simulink model "completo"  (R2014b)
settings: Solver=ode23t  StartTime=0.0  StopTime=10.0  RelTol=1e-3
settings Model: Creator=Javi  LastModifiedBy=Javi

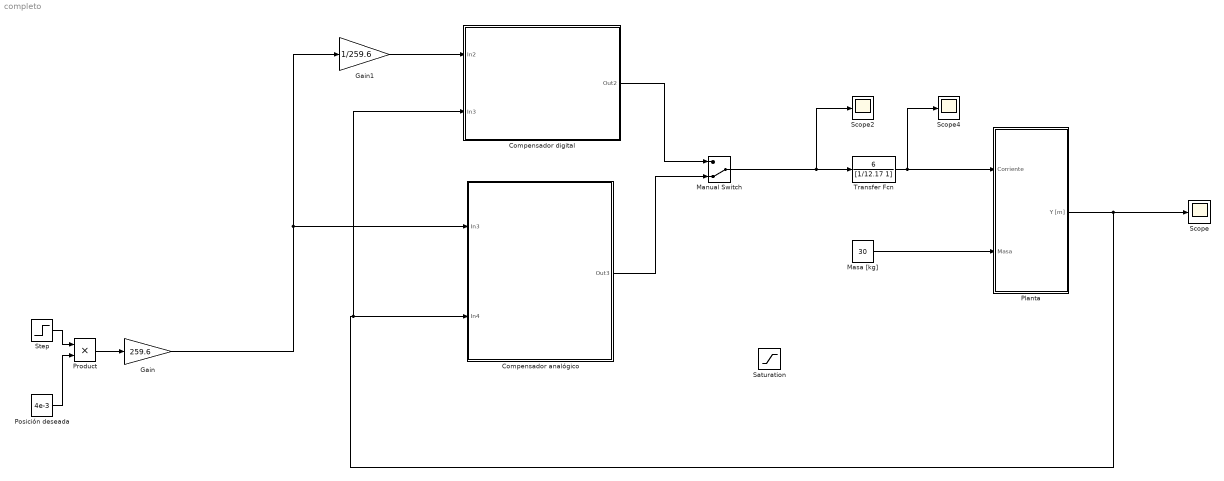
== system completo ==
  Compensador analógico : Subsystem
  Compensador digital : Subsystem
  Gain : Gain  Gain=259.6
  Gain1 : Gain  Gain=1/259.6
  Manual Switch : ManualSwitch  CurrentSetting=0
  "Masa [kg] " : Constant  Value=30
  "Planta " : Subsystem
  Posición deseada : Constant  Value=4e-3
  Product : Product
  Saturation : Saturate  UpperLimit=5  LowerLimit=0
  Scope : Scope
      settings: TimeRange=10  YMin=0  YMax=0.004
  Scope2 : Scope
      settings: TimeRange=10  YMin=-2  YMax=3  SaveName=ScopeData2
  Scope4 : Scope
      settings: TimeRange=0.005185185185185187  YMin=-3500000  YMax=500000  SaveName=ScopeData4
  Step : Step  Time=0.01  SampleTime=0
  Transfer Fcn : TransferFcn  Numerator=[6]  Denominator=[1/12.17 1]
  wires:
  "Masa [kg] "/1 -> "Planta "/2("Masa ")
  "Planta "/1(Y [m]) -> Compensador digital/2(In3), Compensador analógico/2(In4), Scope/1
  Transfer Fcn/1 -> Scope4/1, "Planta "/1(Corriente)
  Step/1 -> Product/1
  Posición deseada/1 -> Product/2
  Product/1 -> Gain/1
  Gain/1 -> Gain1/1, Compensador analógico/1(In3)
  Compensador digital/1(Out2) -> Manual Switch/1
  Compensador analógico/1(Out3) -> Manual Switch/2
  Gain1/1 -> Compensador digital/1(In2)
  Manual Switch/1 -> Scope2/1, Transfer Fcn/1

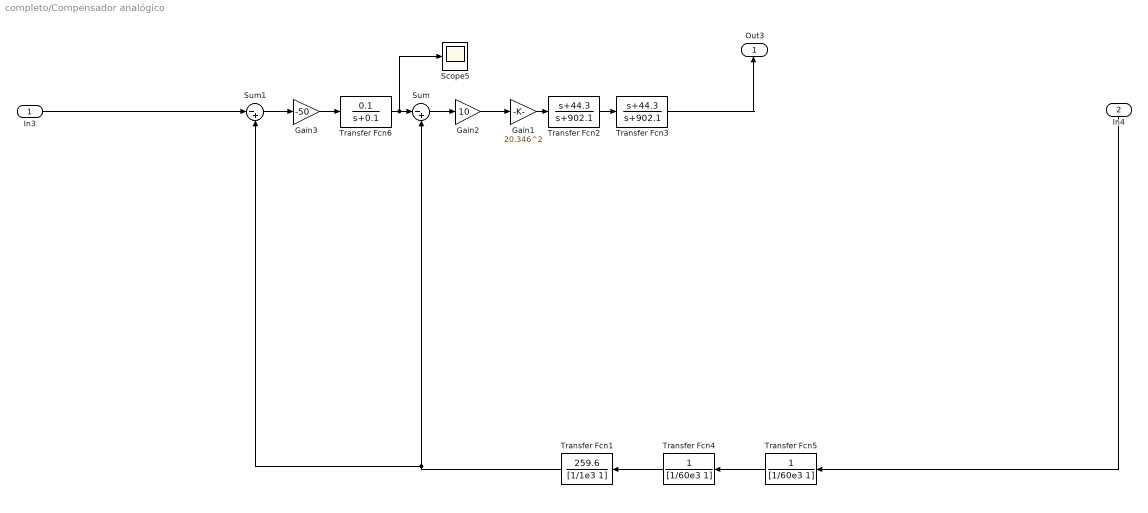
== system completo/Compensador analógico ==
  In3 : Inport
  In4 : Inport  Port=2
  Gain1 : Gain  Gain=20.346^2
  Gain2 : Gain  Gain=10
  Gain3 : Gain  Gain=-50
  Scope5 : Scope
      settings: TimeRange=4  YMin=-0.1  YMax=0.9  SaveName=ScopeData5
  Sum : Sum  Inputs=|-+
  Sum1 : Sum  Inputs=|-+
  Transfer Fcn1 : TransferFcn  Numerator=259.6  Denominator=[1/1e3 1]
  Transfer Fcn2 : TransferFcn  Numerator=[1 44.3]  Denominator=[1 902.1]
  Transfer Fcn3 : TransferFcn  Numerator=[1 44.3]  Denominator=[1 902.1]
  Transfer Fcn4 : TransferFcn  Numerator=1  Denominator=[1/60e3 1]
  Transfer Fcn5 : TransferFcn  Numerator=1  Denominator=[1/60e3 1]
  Transfer Fcn6 : TransferFcn  Numerator=[0.1]  Denominator=[1 0.1]
  Out3 : Outport
  wires:
  Transfer Fcn3/1 -> Out3/1
  Transfer Fcn1/1 -> Sum1/2, Sum/2
  Transfer Fcn2/1 -> Transfer Fcn3/1
  Gain1/1 -> Transfer Fcn2/1
  Sum/1 -> Gain2/1
  Gain2/1 -> Gain1/1
  Transfer Fcn4/1 -> Transfer Fcn1/1
  Transfer Fcn5/1 -> Transfer Fcn4/1
  In4/1 -> Transfer Fcn5/1
  In3/1 -> Sum1/1
  Transfer Fcn6/1 -> Scope5/1, Sum/1
  Gain3/1 -> Transfer Fcn6/1
  Sum1/1 -> Gain3/1

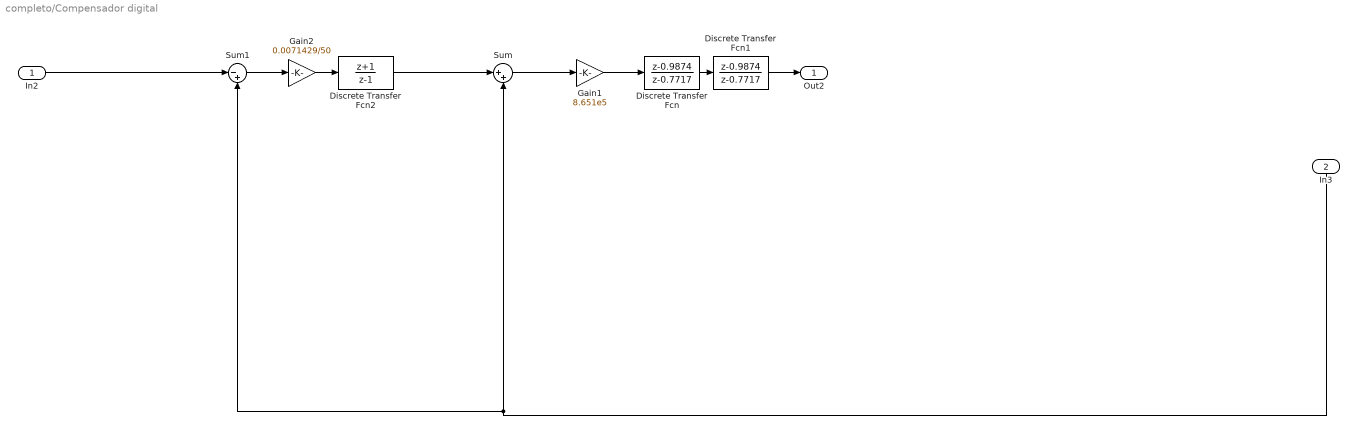
== system completo/Compensador digital ==
  In2 : Inport
  In3 : Inport  Port=2
  Discrete Transfer Fcn : DiscreteTransferFcn  Numerator=[1 -0.9874]  Denominator=[1 -0.7717]  SampleTime=1/3.5e3
  Discrete Transfer Fcn1 : DiscreteTransferFcn  Numerator=[1 -0.9874]  Denominator=[1 -0.7717]
  Discrete Transfer Fcn2 : DiscreteTransferFcn  Numerator=[1 1]  Denominator=[1 -1]  SampleTime=1/3.5e3
  Gain1 : Gain  Gain=8.651e5
  Gain2 : Gain  Gain=0.0071429/50
  Sum : Sum  Inputs=|++
  Sum1 : Sum  Inputs=|-+
  Out2 : Outport
  wires:
  Discrete Transfer Fcn1/1 -> Out2/1
  Sum1/1 -> Gain2/1
  Sum/1 -> Gain1/1
  Discrete Transfer Fcn2/1 -> Sum/1
  In2/1 -> Sum1/1
  Gain1/1 -> Discrete Transfer Fcn/1
  Discrete Transfer Fcn/1 -> Discrete Transfer Fcn1/1
  Gain2/1 -> Discrete Transfer Fcn2/1
  In3/1 -> Sum1/2, Sum/2

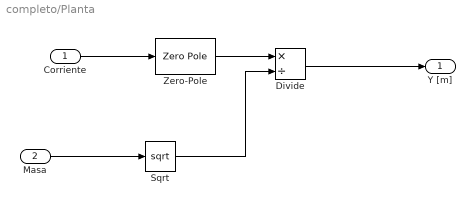
== system completo/Planta  ==
  Corriente : Inport
  "Masa " : Inport  Port=2
  Divide : Product  Inputs=*/
  Sqrt : Sqrt  SaturateOnIntegerOverflow=on
  Zero-Pole : ZeroPole  Zeros=[]  Poles=[70 -70]  Gain=-6.58
  Y [m] : Outport
  wires:
  Divide/1 -> Y [m]/1
  Corriente/1 -> Zero-Pole/1
  Zero-Pole/1 -> Divide/1
  "Masa "/1 -> Sqrt/1
  Sqrt/1 -> Divide/2
